simulink model "D53_LKAS"  (R2018b)
settings: Solver=ode3  StartTime=0.0  StopTime=10.0  FixedStep=0.01  RelTol=1e-3  EnableMultiTasking=on
model workspace (MAT data in the model file):
  MCOS : class17 (value not decoded)
  MCOS : class17 (value not decoded)
  MCOS : class17 (value not decoded)
  MCOS : class17 (value not decoded)
  MCOS : class17 (value not decoded)
  MCOS : class17 (value not decoded)
  MCOS : class17 (value not decoded)
  MCOS : class17 (value not decoded)
  MCOS : class17 (value not decoded)
  MCOS : class17 (value not decoded)
  MCOS : class17 (value not decoded)
  MCOS : class17 (value not decoded)
  MCOS : class17 (value not decoded)
  MCOS : class17 (value not decoded)
  MCOS : class17 (value not decoded)
  MCOS : class17 (value not decoded)
  MCOS : class17 (value not decoded)
  MCOS : class17 (value not decoded)
  MCOS : class17 (value not decoded)
  MCOS : class17 (value not decoded)
  MCOS : class17 (value not decoded)
  MCOS : class17 (value not decoded)
  MCOS : class17 (value not decoded)
  MCOS : class17 (value not decoded)
  MCOS : class17 (value not decoded)
  MCOS : class17 (value not decoded)
  MCOS : class17 (value not decoded)
  MCOS : class17 (value not decoded)
  MCOS : class17 (value not decoded)
  MCOS : class17 (value not decoded)
  MCOS : class17 (value not decoded)
  MCOS : class17 (value not decoded)
  MCOS : class17 (value not decoded)
  MCOS : class17 (value not decoded)
  MCOS : class17 (value not decoded)
  MCOS : class17 (value not decoded)
  MCOS : class17 (value not decoded)
  MCOS : class17 (value not decoded)
  MCOS : class17 (value not decoded)
  MCOS : class17 (value not decoded)
  MCOS : class17 (value not decoded)
  MCOS : class17 (value not decoded)
  MCOS : class17 (value not decoded)
  MCOS : class17 (value not decoded)
  MCOS : class17 (value not decoded)
  MCOS : class17 (value not decoded)
  MCOS : class17 (value not decoded)
  MCOS : class17 (value not decoded)
  MCOS : class17 (value not decoded)
  MCOS : class17 (value not decoded)
  MCOS : class17 (value not decoded)
  MCOS : class17 (value not decoded)
  MCOS : class17 (value not decoded)
  MCOS : class17 (value not decoded)
  MCOS : class17 (value not decoded)
  MCOS : class17 (value not decoded)
  MCOS : class17 (value not decoded)
  MCOS : class17 (value not decoded)
  MCOS : class17 (value not decoded)
  MCOS : class17 (value not decoded)
  MCOS : class17 (value not decoded)
  MCOS : class17 (value not decoded)
  MCOS : class17 (value not decoded)
  MCOS : class17 (value not decoded)
  MCOS : class17 (value not decoded)
  MCOS : class17 (value not decoded)
  MCOS : class17 (value not decoded)
  MCOS : class17 (value not decoded)
  MCOS : class17 (value not decoded)
  MCOS : class17 (value not decoded)
  MCOS : class17 (value not decoded)
  MCOS : class17 (value not decoded)
  MCOS : class17 (value not decoded)
  MCOS : class17 (value not decoded)
  MCOS : class17 (value not decoded)
  MCOS : class17 (value not decoded)
  MCOS : class17 (value not decoded)
  MCOS : class17 (value not decoded)
  MCOS : class17 (value not decoded)
  MCOS : class17 (value not decoded)
  MCOS : class17 (value not decoded)
  MCOS : class17 (value not decoded)
  MCOS : class17 (value not decoded)
  MCOS : class17 (value not decoded)
  MCOS : class17 (value not decoded)
  MCOS : class17 (value not decoded)
  MCOS : class17 (value not decoded)
  MCOS : class17 (value not decoded)
  MCOS : class17 (value not decoded)
values from neighbouring files (symbols this model uses):
  C = who    [Data_Made_Data.m]    (also in Data_Make_Data.m; Data_Process.m)
  LKA_SampleTime = Simulink.Parameter    [Model_NoProtect_Script.m]
  Monitor = find_system(strcat(filename,'/CAN Monitor (CANMon)/Monitor'),'SearchDepth',1,'BlockType','From')    [UpdateMon.m]    (also in UpdateMonAuto.m = find_system(strcat(scriptfile,'/CAN Monitor (CANMon)/Monitor; UpdateMonMdb.m; Update_MonAuto.m = find_system(strcat(scriptfile,'/CAN Monitor (CANMon)/Monitor; Update_MonMdb.m)
undefined symbols (not defined in the file or in its folder): LKA_CarWidth, LKA_StrRatio_C, LKA_Veh2CamL_C, LKA_Veh2CamW_C, LKA_WhlBaseL_C, LL_CompSWA_C, LL_CrvtPrvwT_C, LL_DesDvt_C, LL_DvtComp_C, LL_DvtPrvwT_C, LL_DvtSpdDet_vDvtSpdMin_C, LL_HdAgExT_C, LL_HdAgPrvwT_C, LL_LAccMax_C, LL_LAccRMax_C, LL_LDW_EarliestWarnLine_C, LL_LDW_LatestWarnLine_C, LL_LDWS_SUPPRESS_HEADING, LL_LFClb_TFC_DiffCtlBalance, LL_LFClb_TFC_DiffCtrlMaxSWA, LL_LFClb_TFC_DiffCtrlRatio, LL_LFClb_TFC_facmGainLutGain1_C, LL_LFClb_TFC_facmGainLutGain2_C, LL_LFClb_TFC_facmIntegRatio, LL_LFClb_TFC_facmKlat_C, LL_LFClb_TFC_FfCtlRatio_C, LL_LFClb_TFC_phiIntegCtlMaxSWA_C, LL_LFClb_TFC_tiKlatPrvwT_C, LL_LFClb_TFC_vGainLutVehSpdLwr_C, LL_LFClb_TFC_vGainLutVehSpdUpr_C, LL_LKA_EarliestWarnLine_C, LL_LKA_LatestWarnLine_C, LL_LKAExPrcs_ExitC0Dvt, LL_LKAExPrcs_ExitC0Swt, LL_LKAExPrcs_tiExitTime1, LL_LKAExPrcs_tiExitTime2, LL_LKAExPrcs_tiExitTime3, LL_LKAS_OUT_OF_CONTROL_LAT_VEL, LL_LKAS_OUT_OF_CONTROL_TTLC, LL_LKASWASyn_M0, LL_LKASWASyn_M1, LL_LKASWASyn_M2, LL_LKASWASyn_M3K, LL_LKASWASyn_SWAaddMax, LL_LKASWASyn_T2, LL_LKASWASyn_tiTrqSwaRtTime, LL_LKASWASyn_tiTrqSwaTime, LL_LKASWASyn_TrqMax, LL_LKASWASyn_TrqSwaAddSwt, LL_LKASWASyn_TrqSwaRateDiff, LL_LSpdCompT_C, LL_lStpLngth_C, LL_MAX_DELAY_EPSSTAR_TIME, LL_MAX_DRIVER_TORQUE_DISABLE, LL_MAX_DRIVER_TORQUE_ENABLE, LL_MAX_LANE_WIDTH_DISABLE, LL_MAX_LANE_WIDTH_ENABLE, LL_MAX_LAT_ACC_DISABLE, LL_MAX_LAT_ACC_ENABLE, LL_MAX_LDWS_SPEED_DISABLE ... (+29)
libraries: simulink x134, canmsglib x36, dspstat3 x3, simulink_extras x1
(part 11 of 17)

== system D53_LKAS/LL/LLOn/LKA/LKA Motion Planning (LKAMP) /Motion Planning Input Processing (MPInP)/Lane Information Selection (LaneInfoSel) ==
  LaneInfoSel_stLKAActvFlg : Inport
  LaneInfoSel_facmLftLane : Inport  Port=2
  LaneInfoSel_facmRgtLane : Inport  Port=3
  If : If  IfExpression=u1==1  ElseIfExpressions=u1==2
  If Action Subsystem1 : Subsystem  TreatAsAtomicUnit=on
  If Action Subsystem2 : Subsystem  TreatAsAtomicUnit=on
  If Action Subsystem3 : Subsystem  TreatAsAtomicUnit=on
  Merge : Merge  Inputs=3
  LaneInfoSel_facmActvLane : Outport
  wires:
  If/3 -> If Action Subsystem3/Action
  If Action Subsystem3/1(Out1) -> Merge/3
  If Action Subsystem1/1(Out1) -> Merge/2
  If/2 -> If Action Subsystem1/Action
  Merge/1 -> LaneInfoSel_facmActvLane/1
  If Action Subsystem2/1(Out1) -> Merge/1
  If/1 -> If Action Subsystem2/Action
  LaneInfoSel_stLKAActvFlg/1 -> If/1
  LaneInfoSel_facmLftLane/1 -> If Action Subsystem2/1(In1)
  LaneInfoSel_facmRgtLane/1 -> If Action Subsystem1/1(In1)

== system D53_LKAS/LL/LLOn/LKA/LKA Motion Planning (LKAMP) /Motion Planning Input Processing (MPInP)/Signal Latching2 ==
  In : Inport
  Add : Sum  OutDataTypeStr=uint16
  Constant : Constant  OutDataTypeStr=uint16  SampleTime=-1
  Constant2 : Constant  Value=LatchTime  OutDataTypeStr=uint16  SampleTime=-1
  If : If  NumInputs=2  IfExpression=u1==u2  ShowElse=off
  Memory : Memory  InheritSampleTime=on
  Saturation1 : Saturate  UpperLimit=10000  LowerLimit=0  OutDataTypeStr=uint16
  "if action " : Subsystem  TreatAsAtomicUnit=on
  Out : Outport
  wires:
  Saturation1/1 -> If/1, Memory/1
  Memory/1 -> Add/2
  Add/1 -> Saturation1/1
  Constant/1 -> Add/1
  If/1 -> "if action "/Action
  "if action "/1(Out) -> Out/1
  In/1 -> "if action "/1(In)
  Constant2/1 -> If/2

== system D53_LKAS/LL/LLOn/LKA/LKA Motion Planning (LKAMP) /Motion Planning Input Processing (MPInP)/Signal Latching3 ==
  In : Inport
  Add : Sum  OutDataTypeStr=uint16
  Constant : Constant  OutDataTypeStr=uint16  SampleTime=-1
  Constant2 : Constant  Value=LatchTime  OutDataTypeStr=uint16  SampleTime=-1
  If : If  NumInputs=2  IfExpression=u1==u2  ShowElse=off
  Memory : Memory  InheritSampleTime=on
  Saturation1 : Saturate  UpperLimit=10000  LowerLimit=0  OutDataTypeStr=uint16
  "if action " : Subsystem  TreatAsAtomicUnit=on
  Out : Outport
  wires:
  Constant2/1 -> If/2
  In/1 -> "if action "/1(In)
  "if action "/1(Out) -> Out/1
  If/1 -> "if action "/Action
  Constant/1 -> Add/1
  Add/1 -> Saturation1/1
  Memory/1 -> Add/2
  Saturation1/1 -> Memory/1, If/1

== system D53_LKAS/LL/LLOn/LKA/LKA Motion Planning (LKAMP) /Motion Planning Input Processing (MPInP)/Signal Latching4 ==
  In : Inport
  Add : Sum  OutDataTypeStr=uint16
  Constant : Constant  OutDataTypeStr=uint16  SampleTime=-1
  Constant2 : Constant  Value=LatchTime  OutDataTypeStr=uint16  SampleTime=-1
  If : If  NumInputs=2  IfExpression=u1==u2  ShowElse=off
  Memory : Memory  InheritSampleTime=on
  Saturation1 : Saturate  UpperLimit=10000  LowerLimit=0  OutDataTypeStr=uint16
  "if action " : Subsystem  TreatAsAtomicUnit=on
  Out : Outport
  wires:
  Saturation1/1 -> If/1, Memory/1
  Memory/1 -> Add/2
  Add/1 -> Saturation1/1
  Constant/1 -> Add/1
  If/1 -> "if action "/Action
  "if action "/1(Out) -> Out/1
  In/1 -> "if action "/1(In)
  Constant2/1 -> If/2

== system D53_LKAS/LL/LLOn/LKA/LKA Motion Planning (LKAMP) /Motion Planning Input Processing (MPInP)/Signal Latching5 ==
  In : Inport
  Add : Sum  OutDataTypeStr=uint16
  Constant : Constant  OutDataTypeStr=uint16  SampleTime=-1
  Constant2 : Constant  Value=LatchTime  OutDataTypeStr=uint16  SampleTime=-1
  If : If  NumInputs=2  IfExpression=u1==u2  ShowElse=off
  Memory : Memory  InheritSampleTime=on
  Saturation1 : Saturate  UpperLimit=10000  LowerLimit=0  OutDataTypeStr=uint16
  "if action " : Subsystem  TreatAsAtomicUnit=on
  Out : Outport
  wires:
  Saturation1/1 -> If/1, Memory/1
  Memory/1 -> Add/2
  Add/1 -> Saturation1/1
  Constant/1 -> Add/1
  If/1 -> "if action "/Action
  "if action "/1(Out) -> Out/1
  In/1 -> "if action "/1(In)
  Constant2/1 -> If/2

== system D53_LKAS/LL/LLOn/LKA/LKA Motion Planning (LKAMP) /Motion Planning Input Processing (MPInP)/Signal Latching6 ==
  In : Inport
  Add : Sum  OutDataTypeStr=uint16
  Constant : Constant  OutDataTypeStr=uint16  SampleTime=-1
  Constant2 : Constant  Value=LatchTime  OutDataTypeStr=uint16  SampleTime=-1
  If : If  NumInputs=2  IfExpression=u1==u2  ShowElse=off
  Memory : Memory  InheritSampleTime=on
  Saturation1 : Saturate  UpperLimit=10000  LowerLimit=0  OutDataTypeStr=uint16
  "if action " : Subsystem  TreatAsAtomicUnit=on
  Out : Outport
  wires:
  Saturation1/1 -> If/1, Memory/1
  Memory/1 -> Add/2
  Add/1 -> Saturation1/1
  Constant/1 -> Add/1
  If/1 -> "if action "/Action
  "if action "/1(Out) -> Out/1
  In/1 -> "if action "/1(In)
  Constant2/1 -> If/2

== system D53_LKAS/LL/LLOn/LKA/LKA Motion Planning (LKAMP) /Motion Planning Input Processing (MPInP)/Signal Latching7 ==
  In : Inport
  Add : Sum  OutDataTypeStr=uint16
  Constant : Constant  OutDataTypeStr=uint16  SampleTime=-1
  Constant2 : Constant  Value=LatchTime  OutDataTypeStr=uint16  SampleTime=-1
  If : If  NumInputs=2  IfExpression=u1==u2  ShowElse=off
  Memory : Memory  InheritSampleTime=on
  Saturation1 : Saturate  UpperLimit=10000  LowerLimit=0  OutDataTypeStr=uint16
  "if action " : Subsystem  TreatAsAtomicUnit=on
  Out : Outport
  wires:
  Constant2/1 -> If/2
  In/1 -> "if action "/1(In)
  "if action "/1(Out) -> Out/1
  If/1 -> "if action "/Action
  Constant/1 -> Add/1
  Add/1 -> Saturation1/1
  Memory/1 -> Add/2
  Saturation1/1 -> Memory/1, If/1

== system D53_LKAS/LL/LLOn/LKA/LKA Motion Planning (LKAMP) /Motion Planning Input Processing (MPInP)/Subsystem ==
  In1 : Inport
  If : If  IfExpression=u1==1  ElseIfExpressions=u1==2
  If Action Subsystem1 : Subsystem  TreatAsAtomicUnit=on
  If Action Subsystem2 : Subsystem  TreatAsAtomicUnit=on
  If Action Subsystem3 : Subsystem  TreatAsAtomicUnit=on
  Merge : Merge  Inputs=3
  Out6 : Outport
  wires:
  In1/1 -> If/1
  If/1 -> If Action Subsystem2/Action
  If Action Subsystem2/1(Out1) -> Merge/1
  Merge/1 -> Out6/1
  If/2 -> If Action Subsystem1/Action
  If Action Subsystem1/1(Out1) -> Merge/2
  If Action Subsystem3/1(Out1) -> Merge/3
  If/3 -> If Action Subsystem3/Action

== system D53_LKAS/LL/LLOn/LKA/LKA Motion Planning (LKAMP) /Switching Condition (SwtCon)/Ending Heading Angle Determination (EndHdAgDet) ==
  EndHdAgDet_stLKAActvFlg : Inport
  EndHdAgDet_vVehSpd : Inport  Port=2
  EndHdAgDet_crPrvwCrvt : Inport  Port=3
  EndHdAgDet_lLaneWidth_C : Inport  Port=4
  EndHdAgDet_lCarWidth_C : Inport  Port=5
  EndHdAgDet_tiHdAgExTime_C : Inport  Port=6
  EndHdAgDet_tiLSpdCompT_C : Inport  Port=7
  Add : Sum  Inputs=+-  OutDataTypeStr=single
  Add1 : Sum  OutDataTypeStr=single
  Divide : Product  Inputs=/*  OutDataTypeStr=single
  Divide1 : Product  Inputs=*/  OutDataTypeStr=single
  Lateral Speed Compensation (LSpdComp) : Subsystem
  kph To mps : Gain  Gain=1/3.6  OutDataTypeStr=single
  EndHdAgDet_phiHdAgMax : Outport
  wires:
  Divide/1 -> Divide1/1
  EndHdAgDet_lLaneWidth_C/1 -> Add/1
  EndHdAgDet_lCarWidth_C/1 -> Add/2
  kph To mps/1 -> Lateral Speed Compensation (LSpdComp)/1(LSpdComp_vVehSpd), Divide1/2
  EndHdAgDet_tiHdAgExTime_C/1 -> Divide/1
  EndHdAgDet_vVehSpd/1 -> kph To mps/1
  EndHdAgDet_stLKAActvFlg/1 -> Lateral Speed Compensation (LSpdComp)/2(LSpdComp_stLKAFlg)
  Add/1 -> Divide/2
  Lateral Speed Compensation (LSpdComp)/1(LSpdComp_phiLSpdComp) -> Add1/2
  Divide1/1 -> Add1/1
  Add1/1 -> EndHdAgDet_phiHdAgMax/1
  EndHdAgDet_crPrvwCrvt/1 -> Lateral Speed Compensation (LSpdComp)/3(LSpdComp_crPrvwCrvt)
  EndHdAgDet_tiLSpdCompT_C/1 -> Lateral Speed Compensation (LSpdComp)/4(LSpdComp_tiLSpdCompT_C)

== system D53_LKAS/LL/LLOn/LKA/LKA Motion Planning (LKAMP) /Switching Condition (SwtCon)/If Action Subsystem ==
  In1 : Inport
  Action Port : ActionPort  InitializeStates=reset
  Gain2 : Gain  Gain=-1  OutDataTypeStr=Inherit: Same as input
  Out1 : Outport
  wires:
  Gain2/1 -> Out1/1  "HdAgMax"
  In1/1 -> Gain2/1

== system D53_LKAS/LL/LLOn/LKA/LKA Motion Planning (LKAMP) /Switching Condition (SwtCon)/If Action Subsystem1 ==
  In1 : Inport
  Action Port : ActionPort  InitializeStates=reset
  Cast To Single1 : DataTypeConversion  LockScale=on
  Out1 : Outport
  wires:
  Cast To Single1/1 -> Out1/1  "HdAgMax"
  In1/1 -> Cast To Single1/1

== system D53_LKAS/LL/LLOn/LKA/LKA Motion Planning (LKAMP) /Switching Condition (SwtCon)/If Action Subsystem2 ==
  Action Port : ActionPort  InitializeStates=reset
  Constant2 : Constant  Value=0  OutDataTypeStr=single  SampleTime=-1
  Out1 : Outport
  wires:
  Constant2/1 -> Out1/1  "HdAgMax"

== system D53_LKAS/LL/LLOn/LKA/LKA Motion Planning (LKAMP) /Switching Condition (SwtCon)/Signal Latching ==
  In : Inport
  Add : Sum  OutDataTypeStr=uint16
  Constant : Constant  OutDataTypeStr=uint16  SampleTime=-1
  Constant2 : Constant  Value=LatchTime  OutDataTypeStr=uint16  SampleTime=-1
  If : If  NumInputs=2  IfExpression=u1==u2  ShowElse=off
  Memory : Memory  InheritSampleTime=on
  Saturation1 : Saturate  UpperLimit=10000  LowerLimit=0  OutDataTypeStr=uint16
  "if action " : Subsystem  TreatAsAtomicUnit=on
  Out : Outport
  wires:
  Saturation1/1 -> If/1
  Memory/1 -> Add/2
  Add/1 -> Saturation1/1, Memory/1
  Constant/1 -> Add/1
  If/1 -> "if action "/Action
  "if action "/1(Out) -> Out/1
  In/1 -> "if action "/1(In)
  Constant2/1 -> If/2

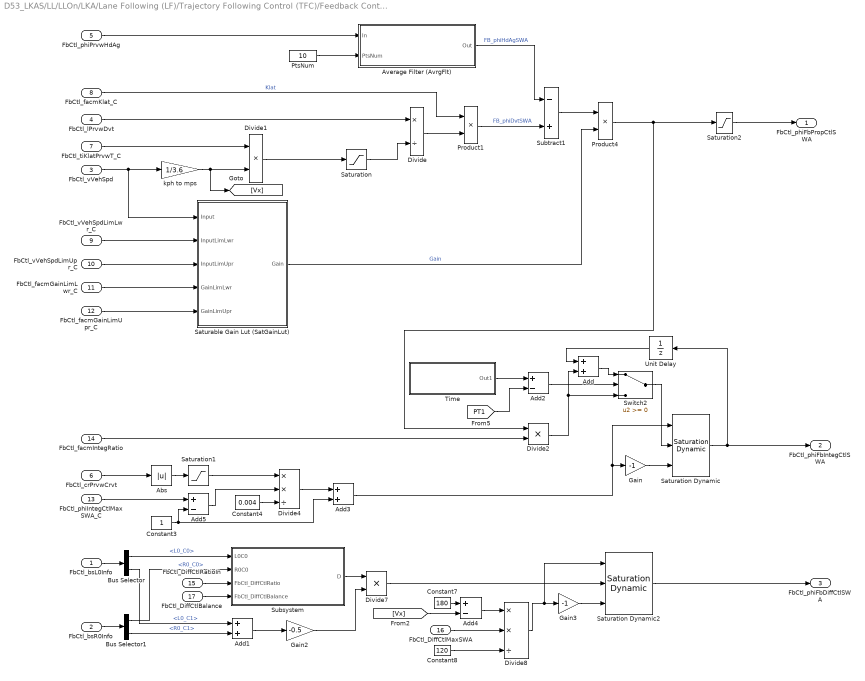
== system D53_LKAS/LL/LLOn/LKA/Lane Following (LF)/Trajectory Following Control (TFC)/Feedback Control (FbCtl) ==
  FbCtl_bsL0Info : Inport
  FbCtl_bsR0Info : Inport  Port=2
  FbCtl_vVehSpd : Inport  Port=3
  FbCtl_lPrvwDvt : Inport  Port=4
  FbCtl_phiPrvwHdAg : Inport  Port=5
  FbCtl_crPrvwCrvt : Inport  Port=6
  FbCtl_tiKlatPrvwT_C : Inport  Port=7
  FbCtl_facmKlat_C : Inport  Port=8
  FbCtl_vVehSpdLimLwr_C : Inport  Port=9
  FbCtl_vVehSpdLimUpr_C : Inport  Port=10
  FbCtl_facmGainLimLwr_C : Inport  Port=11
  FbCtl_facmGainLimUpr_C : Inport  Port=12
  FbCtl_phiIntegCtlMaxSWA_C : Inport  Port=13
  FbCtl_facmIntegRatio : Inport  Port=14
  FbCtl_DiffCtlRatioIn : Inport  Port=15
  FbCtl_DiffCtlMaxSWA : Inport  Port=16
  FbCtl_DiffCtlBalance : Inport  Port=17
  Abs : Abs
  Add : Sum
  Add1 : Sum
  Add2 : Sum  Inputs=+-
  Add3 : Sum
  Add4 : Sum  Inputs=+-
  Add5 : Sum  Inputs=+-
  Average Filter (AvrgFlt) : Subsystem
      mask Display:
      | port_label('input', 1, 'In');
      | port_label('input', 2, 'PtsNum');
      | port_label('output', 1, 'Out');
      | color('blue');
      | text(0.98,0.9,'VCDC Block','horizontalAlignment','right');
      | color('black');
      | text(0.5,0.55,'Average Filter','horizontalAlignment','center');
      | text(0.5,0.4,'(AvrgFlt)','horizontalAlignment','center');
  Bus Selector : BusSelector  OutputSignals=L0_C0,L0_C1
  Bus Selector1 : BusSelector  OutputSignals=R0_C0,R0_C1
  Constant3 : Constant  OutDataTypeStr=single
  Constant4 : Constant  Value=0.004  OutDataTypeStr=single
  Constant7 : Constant  Value=180  OutDataTypeStr=single
  Constant8 : Constant  Value=120  OutDataTypeStr=single
  Divide : Product  Inputs=*/
  Divide1 : Product  Inputs=**
  Divide2 : Product  Inputs=**
  Divide4 : Product  Inputs=**/
  Divide7 : Product  Inputs=**
  Divide8 : Product  Inputs=**/
  Gain : Gain  Gain=-1  OutDataTypeStr=single
  Gain2 : Gain  Gain=-0.5
  Gain3 : Gain  Gain=-1  OutDataTypeStr=single
  Product1 : Product  OutDataTypeStr=single  RndMeth=Zero
  Product4 : Product  OutDataTypeStr=single  RndMeth=Zero
  PtsNum : Constant  Value=10  OutDataTypeStr=single
  Saturable Gain Lut (SatGainLut) : MATLAB Function  TreatAsAtomicUnit=on
  Saturation : Saturate  UpperLimit=40  LowerLimit=5
  Saturation Dynamic : simulink/Discontinuities/Saturation Dynamic  OutMin=[]  OutMax=[]  OutDataTypeStr=Inherit: Same as second input  OutDataType=fixdt(1, 16)  OutScaling=2^-10  DoSatur=off
  Saturation Dynamic2 : simulink/Discontinuities/Saturation Dynamic  OutMin=[]  OutMax=[]  OutDataTypeStr=Inherit: Same as second input  OutDataType=fixdt(1, 16)  OutScaling=2^-10  DoSatur=off
  Saturation1 : Saturate  UpperLimit=0.004  LowerLimit=0.00001
  Saturation2 : Saturate  UpperLimit=360  LowerLimit=-360  OutDataTypeStr=single
  Subsystem : Subsystem
  Subtract1 : Sum  Inputs=-+
  Switch2 : Switch
  Time : Subsystem
      mask Display:
      | port_label('output', 1, 'TTime');
      | color('blue');
      | text(0.98,0.9,'VCDC Block','horizontalAlignment','right');
      | color('black');
      | text(0.5,0.55,'Tick Time','horizontalAlignment','center');
      | text(0.5,0.4,'(TTime)','horizontalAlignment','center');
  Unit Delay : UnitDelay  SampleTime=-1
  kph to mps : Gain  Gain=1/3.6  OutDataTypeStr=single
  FbCtl_phiFbPropCtlSWA : Outport
  FbCtl_phiFbIntegCtlSWA : Outport  Port=2
  FbCtl_phiFbDiffCtlSWA : Outport  Port=3
  wires:
  FbCtl_DiffCtlBalance/1 -> Subsystem/4(FbCtl_DiffCtlBalance)
  Add5/1 -> Divide4/2
  Constant4/1 -> Divide4/3
  Divide4/1 -> Add3/1
  Saturation1/1 -> Divide4/1
  Constant3/1 -> Add3/2, Add5/2
  Abs/1 -> Saturation1/1
  FbCtl_crPrvwCrvt/1 -> Abs/1
  Add/1 -> Switch2/1
  Switch2/1 -> Saturation Dynamic/2
  Add2/1 -> Switch2/2
  [PT1] -> Add2/2
  Time/1(Out1) -> Add2/1
  Saturation Dynamic2/1 -> FbCtl_phiFbDiffCtlSWA/1
  FbCtl_DiffCtlRatioIn/1 -> Subsystem/3(FbCtl_DiffCtlRatio)
  Subsystem/1(D) -> Divide7/1
  Bus Selector1/2 -> Add1/2  "<R0_C1>"
  Add1/1 -> Gain2/1
  Bus Selector/2 -> Add1/1  "<L0_C1>"
  [Vx] -> Add4/2
  Constant8/1 -> Divide8/3
  Add4/1 -> Divide8/1
  Constant7/1 -> Add4/1
  FbCtl_DiffCtlMaxSWA/1 -> Divide8/2
  Divide8/1 -> Saturation Dynamic2/1, Gain3/1
  Gain3/1 -> Saturation Dynamic2/3
  Divide7/1 -> Saturation Dynamic2/2
  Saturation Dynamic/1 -> Unit Delay/1, FbCtl_phiFbIntegCtlSWA/1
  Gain/1 -> Saturation Dynamic/3
  Unit Delay/1 -> Add/1
  FbCtl_vVehSpd/1 -> Saturable Gain Lut (SatGainLut)/1(Input), kph to mps/1
  FbCtl_phiIntegCtlMaxSWA_C/1 -> Add5/1
  Add3/1 -> Gain/1, Saturation Dynamic/1
  Subtract1/1 -> Product4/1
  Divide2/1 -> Switch2/3, Add/2
  FbCtl_facmIntegRatio/1 -> Divide2/2
  FbCtl_facmGainLimUpr_C/1 -> Saturable Gain Lut (SatGainLut)/5(GainLimUpr)
  FbCtl_facmGainLimLwr_C/1 -> Saturable Gain Lut (SatGainLut)/4(GainLimLwr)
  FbCtl_vVehSpdLimUpr_C/1 -> Saturable Gain Lut (SatGainLut)/3(InputLimUpr)
  FbCtl_vVehSpdLimLwr_C/1 -> Saturable Gain Lut (SatGainLut)/2(InputLimLwr)
  kph to mps/1 -> [Vx], Divide1/2
  Product4/1 -> Saturation2/1, Divide2/1
  FbCtl_phiPrvwHdAg/1 -> Average Filter (AvrgFlt)/1(In)
  Divide/1 -> Product1/2
  FbCtl_lPrvwDvt/1 -> Divide/1
  FbCtl_tiKlatPrvwT_C/1 -> Divide1/1
  Divide1/1 -> Saturation/1
  Saturation/1 -> Divide/2
  Saturation2/1 -> FbCtl_phiFbPropCtlSWA/1
  Saturable Gain Lut (SatGainLut)/1(Gain) -> Product4/2  "Gain"
  Average Filter (AvrgFlt)/1(Out) -> Subtract1/1  "FB_phiHdAgSWA"
  Product1/1 -> Subtract1/2  "FB_phiDvtSWA"
  FbCtl_facmKlat_C/1 -> Product1/1  "Klat"
  PtsNum/1 -> Average Filter (AvrgFlt)/2(PtsNum)
  FbCtl_bsL0Info/1 -> Bus Selector/1
  FbCtl_bsR0Info/1 -> Bus Selector1/1
  Bus Selector/1 -> Subsystem/1(L0C0)  "<L0_C0>"
  Bus Selector1/1 -> Subsystem/2(R0C0)  "<R0_C0>"
  Gain2/1 -> Divide7/2

== system D53_LKAS/LL/LLOn/LKA/Lane Following (LF)/Trajectory Following Control (TFC)/Feedforward Control (FfCtl) ==
  FfCtl_FfCtlRatio_C : Inport
  FfCtl_vVehSpd : Inport  Port=2
  FfCtl_crPrvwCrvt : Inport  Port=3
  FfCtl_lWhlBase_SY : Inport  Port=4
  FfCtl_rTraRatio_C : Inport  Port=5
  Add : Sum  OutDataTypeStr=single
  Constant1 : Constant  OutDataTypeStr=single
  Divide : Product  Inputs=*/  OutDataTypeStr=single
  Divide1 : Product  Inputs=*/  OutDataTypeStr=single
  Gain2 : Gain  Gain=-1  OutDataTypeStr=single
  Lookup Table2 : Lookup_n-D  NumberOfTableDimensions=1  BreakpointsForDimension1=[11.7,18.83,26.98,31.98,51.04,79,86.08,90.59]  BeginIndexSearchUsingPreviousIndexResult=on  Table=[0.012141,0.005179,0.00298,0.002547,0.001715,0.001283,0.001021,0.000982]  DiagnosticForOutOfRangeInput=Warning  RemoveProtectionInput=on  InternalRulePriority=Speed  OutDataTypeStr=single  InputSameDT=on
  Math Function : Math  Operator=magnitude^2  OutDataTypeStr=single  SaturateOnIntegerOverflow=on
  Product : Product  OutDataTypeStr=single
  Product1 : Product  OutDataTypeStr=single
  Product2 : Product  OutDataTypeStr=single
  Product3 : Product  Inputs=3  OutDataTypeStr=single
  Saturation1 : Saturate  UpperLimit=0.01  LowerLimit=0
  kph to mps : Gain  Gain=1/3.6  OutDataTypeStr=single
  rad to deg : Gain  Gain=180/pi  OutDataTypeStr=single
  FfCtl_phiFfSWA : Outport
  wires:
  Saturation1/1 -> Product2/2  "FfCtl_facmUSG_C"
  Lookup Table2/1 -> Saturation1/1
  FfCtl_FfCtlRatio_C/1 -> Product3/1
  FfCtl_rTraRatio_C/1 -> Product3/3
  Product3/1 -> Gain2/1
  FfCtl_vVehSpd/1 -> kph to mps/1, Lookup Table2/1
  FfCtl_crPrvwCrvt/1 -> Product/2
  Product/1 -> rad to deg/1
  Math Function/1 -> Product2/1
  Product2/1 -> Add/1
  Constant1/1 -> Add/2
  Add/1 -> Divide1/1
  FfCtl_lWhlBase_SY/1 -> Divide/2
  Divide/1 -> Divide1/2
  Divide1/1 -> Product1/2
  Product1/1 -> Product3/2
  rad to deg/1 -> Product1/1
  kph to mps/1 -> Product/1, Math Function/1, Divide/1
  Gain2/1 -> FfCtl_phiFfSWA/1

== system D53_LKAS/LL/LLOn/LKA/Plan To LaneFollowing (PTLF)/InsideJudge1/If Action Subsystem ==
  T1 : Inport
  Plan : Inport  Port=2
  HdAgLft : Inport  Port=3
  Time : Inport  Port=4
  Action Port : ActionPort  InitializeStates=reset
  Add : Sum
  Cast To Single : DataTypeConversion  OutDataTypeStr=uint8
  Compare To Constant : simulink/Logic and Bit Operations/Compare To Constant  relop=>=  const=0  OutDataTypeStr=boolean
  Detect Decrease : simulink/Logic and Bit Operations/Detect Decrease  vinit=0.0  OutDataTypeStr=boolean
  If Action Subsystem : Subsystem  TreatAsAtomicUnit=on
  If Action Subsystem2 : Subsystem  TreatAsAtomicUnit=on
  Logical Operator : Logic  AllPortsSameDT=off  OutDataTypeStr=boolean
  Memory : Memory  InheritSampleTime=on
  Relational Operator : RelationalOperator  OutDataTypeStr=boolean  RndMeth=Simplest
  Saturation : Saturate  UpperLimit=5  LowerLimit=0
  Switch : Switch  Criteria=u2 > Threshold
  Switch1 : Switch  Criteria=u2 > Threshold
  T1_1 : Outport
  Plan_1 : Outport  Port=2
  wires:
  Switch1/1 -> Plan_1/1
  Switch/1 -> T1_1/1
  If Action Subsystem2/2(Plan_1) -> Switch1/3
  If Action Subsystem2/1(T1_1) -> Switch/3
  If Action Subsystem/2(Plan_1) -> Switch1/1
  If Action Subsystem/1(T1_1) -> Switch/1
  Saturation/1 -> Memory/1, If Action Subsystem/Enable, Switch/2, Switch1/2
  Cast To Single/1 -> Add/1
  Logical Operator/1 -> Cast To Single/1
  Memory/1 -> Add/2
  Add/1 -> Saturation/1
  Relational Operator/1 -> Logical Operator/2
  Detect Decrease/1 -> Logical Operator/1
  T1/1 -> Relational Operator/1, If Action Subsystem2/1(T1)
  Plan/1 -> If Action Subsystem/2(Plan), If Action Subsystem2/2(Plan)
  Time/1 -> Relational Operator/2, If Action Subsystem/1(T1)
  Compare To Constant/1 -> Detect Decrease/1
  HdAgLft/1 -> Compare To Constant/1

== system D53_LKAS/LL/LLOn/LKA/Plan To LaneFollowing (PTLF)/InsideJudge1/If Action Subsystem1 ==
  T1 : Inport
  Plan : Inport  Port=2
  HdAgRgt : Inport  Port=3
  Time : Inport  Port=4
  Action Port : ActionPort  InitializeStates=reset
  Add : Sum
  Cast To Single : DataTypeConversion  OutDataTypeStr=uint8
  Compare To Constant : simulink/Logic and Bit Operations/Compare To Constant  relop=<=  const=0  OutDataTypeStr=boolean
  Detect Decrease : simulink/Logic and Bit Operations/Detect Decrease  vinit=0.0  OutDataTypeStr=boolean
  If Action Subsystem : Subsystem  TreatAsAtomicUnit=on
  If Action Subsystem2 : Subsystem  TreatAsAtomicUnit=on
  Logical Operator : Logic  AllPortsSameDT=off  OutDataTypeStr=boolean
  Memory : Memory  InheritSampleTime=on
  Relational Operator : RelationalOperator  OutDataTypeStr=boolean  RndMeth=Simplest
  Saturation : Saturate  UpperLimit=5  LowerLimit=0
  Switch : Switch  Criteria=u2 > Threshold
  Switch1 : Switch  Criteria=u2 > Threshold
  T1_1 : Outport
  Plan_1 : Outport  Port=2
  wires:
  Plan/1 -> If Action Subsystem2/2(Plan), If Action Subsystem/2(Plan)
  If Action Subsystem/1(T1_1) -> Switch/1
  If Action Subsystem2/2(Plan_1) -> Switch1/3
  Switch1/1 -> Plan_1/1
  Switch/1 -> T1_1/1
  If Action Subsystem/2(Plan_1) -> Switch1/1
  If Action Subsystem2/1(T1_1) -> Switch/3
  Saturation/1 -> If Action Subsystem/Enable, Switch/2, Switch1/2, Memory/1
  Cast To Single/1 -> Add/1
  Logical Operator/1 -> Cast To Single/1
  Memory/1 -> Add/2
  T1/1 -> Relational Operator/1, If Action Subsystem2/1(T1)
  Add/1 -> Saturation/1
  Time/1 -> If Action Subsystem/1(T1), Relational Operator/2
  HdAgRgt/1 -> Compare To Constant/1
  Compare To Constant/1 -> Detect Decrease/1
  Detect Decrease/1 -> Logical Operator/1
  Relational Operator/1 -> Logical Operator/2

== system D53_LKAS/LL/LLOn/LKA/Plan To LaneFollowing (PTLF)/InsideJudge1/If Action Subsystem2 ==
  T1 : Inport
  Plan : Inport  Port=2
  Action Port : ActionPort  InitializeStates=reset
  T1_1 : Outport
  Plan_1 : Outport  Port=2
  wires:
  Plan/1 -> Plan_1/1
  T1/1 -> T1_1/1

== system D53_LKAS/LL/LLOn/LKA Input Processing (LKAInP)/Predicted Deviation Calculation (PrDvt)/Lane Information Selection (LaneInfoSel)/If Action Subsystem1 ==
  In1 : Inport
  Action Port : ActionPort  InitializeStates=reset
  Out1 : Outport
  wires:
  In1/1 -> Out1/1

== system D53_LKAS/LL/LLOn/LKA Input Processing (LKAInP)/Predicted Deviation Calculation (PrDvt)/Lane Information Selection (LaneInfoSel)/If Action Subsystem2 ==
  In1 : Inport
  Action Port : ActionPort  InitializeStates=reset
  Out1 : Outport
  wires:
  In1/1 -> Out1/1

== system D53_LKAS/LL/LLOn/LKA Input Processing (LKAInP)/Predicted Deviation Calculation (PrDvt)/Lane Information Selection (LaneInfoSel)/If Action Subsystem3 ==
  In1 : Inport
  In2 : Inport  Port=2
  Action Port : ActionPort  InitializeStates=reset
  Add : Sum
  Gain : Gain  Gain=0.5
  Out1 : Outport
  wires:
  Add/1 -> Gain/1
  In2/1 -> Add/2
  In1/1 -> Add/1
  Gain/1 -> Out1/1

== system D53_LKAS/LL/LLOn/LKA Input Processing (LKAInP)/Predicted Deviation Calculation (PrDvt)/Lane Information Selection (LaneInfoSel)1/If Action Subsystem1 ==
  In1 : Inport
  Action Port : ActionPort  InitializeStates=reset
  Out1 : Outport
  wires:
  In1/1 -> Out1/1

== system D53_LKAS/LL/LLOn/LKA Input Processing (LKAInP)/Predicted Deviation Calculation (PrDvt)/Lane Information Selection (LaneInfoSel)1/If Action Subsystem2 ==
  In1 : Inport
  Action Port : ActionPort  InitializeStates=reset
  Out1 : Outport
  wires:
  In1/1 -> Out1/1

== system D53_LKAS/LL/LLOn/LKA Input Processing (LKAInP)/Predicted Deviation Calculation (PrDvt)/Lane Information Selection (LaneInfoSel)1/If Action Subsystem3 ==
  In1 : Inport
  In2 : Inport  Port=2
  Action Port : ActionPort  InitializeStates=reset
  Min : MinMax  Inputs=2
  Out1 : Outport
  wires:
  Min/1 -> Out1/1
  In1/1 -> Min/1
  In2/1 -> Min/2

== system D53_LKAS/LL/LLOn/LKA Input Processing (LKAInP)/Predicted Heading Angle Calculation (PrHdAg)/Lane Information Selection (LaneInfoSel)/If Action Subsystem1 ==
  In1 : Inport
  Action Port : ActionPort  InitializeStates=reset
  Out1 : Outport
  wires:
  In1/1 -> Out1/1

== system D53_LKAS/LL/LLOn/LKA Input Processing (LKAInP)/Predicted Heading Angle Calculation (PrHdAg)/Lane Information Selection (LaneInfoSel)/If Action Subsystem2 ==
  In1 : Inport
  Action Port : ActionPort  InitializeStates=reset
  Out1 : Outport
  wires:
  In1/1 -> Out1/1

== system D53_LKAS/LL/LLOn/LKA Input Processing (LKAInP)/Predicted Heading Angle Calculation (PrHdAg)/Lane Information Selection (LaneInfoSel)/If Action Subsystem3 ==
  In1 : Inport
  In2 : Inport  Port=2
  Action Port : ActionPort  InitializeStates=reset
  Add : Sum
  Gain : Gain  Gain=0.5
  Out1 : Outport
  wires:
  In2/1 -> Add/2
  In1/1 -> Add/1
  Add/1 -> Gain/1
  Gain/1 -> Out1/1

== system D53_LKAS/LL/LLOn/LKA Input Processing (LKAInP)/Predicted Heading Angle Calculation (PrHdAg)/Lane Information Selection (LaneInfoSel)1/If Action Subsystem1 ==
  In1 : Inport
  Action Port : ActionPort  InitializeStates=reset
  Out1 : Outport
  wires:
  In1/1 -> Out1/1

== system D53_LKAS/LL/LLOn/LKA Input Processing (LKAInP)/Predicted Heading Angle Calculation (PrHdAg)/Lane Information Selection (LaneInfoSel)1/If Action Subsystem2 ==
  In1 : Inport
  Action Port : ActionPort  InitializeStates=reset
  Out1 : Outport
  wires:
  In1/1 -> Out1/1

== system D53_LKAS/LL/LLOn/LKA Input Processing (LKAInP)/Predicted Heading Angle Calculation (PrHdAg)/Lane Information Selection (LaneInfoSel)1/If Action Subsystem3 ==
  In1 : Inport
  In2 : Inport  Port=2
  Action Port : ActionPort  InitializeStates=reset
  Add : Sum
  Gain : Gain  Gain=0.5
  Out1 : Outport
  wires:
  Gain/1 -> Out1/1
  Add/1 -> Gain/1
  In1/1 -> Add/1
  In2/1 -> Add/2

== system D53_LKAS/LL/LLOn/LKA Input Processing (LKAInP)/Predicted Heading Angle Calculation (PrHdAg)/Perdicted Heading Angle Compensation (PrdcHdAgComp)/Yaw Rate Stable Gain (YRSG) ==
  YRSG_vVehSpd : Inport
  Add : Sum  OutDataTypeStr=single
  Bus Selector : BusSelector  OutputSignals=LKA_WhlBaseL_C
  Divide2 : Product  Inputs=*/  OutDataTypeStr=single
  Divide3 : Product  Inputs=*/  OutDataTypeStr=single
  Lookup Table2 : Lookup_n-D  NumberOfTableDimensions=1  BreakpointsForDimension1=[11.7,18.83,26.98,31.98,51.04,79,86.08,90.59]  BeginIndexSearchUsingPreviousIndexResult=on  Table=[0.012141,0.005179,0.00298,0.002547,0.001715,0.001283,0.001021,0.000982]  DiagnosticForOutOfRangeInput=Warning  RemoveProtectionInput=on  InternalRulePriority=Speed  OutDataTypeStr=single  InputSameDT=on
  Product1 : Product  Inputs=3  OutDataTypeStr=single
  Saturation1 : Saturate  UpperLimit=0.012141  LowerLimit=0.000982
  "constant " : Constant  OutDataTypeStr=single
  kph To mps : Gain  Gain=1/3.6  OutDataTypeStr=single
  YRSG_dphiYRSG : Outport
  wires:
  [LLClb_bsConstantClb] -> Bus Selector/1
  YRSG_vVehSpd/1 -> kph To mps/1, Lookup Table2/1
  Bus Selector/1 -> Divide2/2  "<LKA_WhlBaseL_C>"
  Divide2/1 -> Divide3/1
  Product1/1 -> Add/1
  "constant "/1 -> Add/2
  Add/1 -> Divide3/2
  Divide3/1 -> YRSG_dphiYRSG/1
  Lookup Table2/1 -> Saturation1/1
  Saturation1/1 -> Product1/3
  kph To mps/1 -> Product1/2, Product1/1, Divide2/1

== system D53_LKAS/LL/LLOn/LKA Input Processing (LKAInP)/Previewed Curvature (PrCrvt)/Lane Information Selection (LaneInfoSel)/If Action Subsystem1 ==
  In1 : Inport
  Action Port : ActionPort  InitializeStates=reset
  Out1 : Outport
  wires:
  In1/1 -> Out1/1

== system D53_LKAS/LL/LLOn/LKA Input Processing (LKAInP)/Previewed Curvature (PrCrvt)/Lane Information Selection (LaneInfoSel)/If Action Subsystem2 ==
  In1 : Inport
  Action Port : ActionPort  InitializeStates=reset
  Out1 : Outport
  wires:
  In1/1 -> Out1/1

== system D53_LKAS/LL/LLOn/LKA Input Processing (LKAInP)/Previewed Curvature (PrCrvt)/Lane Information Selection (LaneInfoSel)/If Action Subsystem3 ==
  In1 : Inport
  In2 : Inport  Port=2
  Action Port : ActionPort  InitializeStates=reset
  Add : Sum
  Gain : Gain  Gain=0.5
  Out1 : Outport
  wires:
  Add/1 -> Gain/1
  In2/1 -> Add/2
  In1/1 -> Add/1
  Gain/1 -> Out1/1

== system D53_LKAS/LL/LLOn/LKA Input Processing (LKAInP)/Steering Wheel Position Calculation (SWAPosCal)/Subsystem/LowPass ==
  T : Inport
  u : Inport  Port=2
  dT : Inport  Port=3
  Add : Sum  Inputs=+-
  Add1 : Sum
  Add2 : Sum  OutDataTypeStr=single
  Divide : Product  Inputs=*/
  Divide1 : Product  Inputs=**
  Memory3 : Memory  InheritSampleTime=on
  SWACmdSyn_tiSmplT_C4 : Constant  OutDataTypeStr=single
  Saturation : Saturate  UpperLimit=50  LowerLimit=0
  Switch : Switch  Criteria=u2 > Threshold  Threshold=1
  Unit Delay : UnitDelay  SampleTime=-1
  y : Outport
  wires:
  T/1 -> Divide/2
  dT/1 -> Divide/1
  u/1 -> Switch/3, Add/1
  Divide/1 -> Divide1/1
  Add/1 -> Divide1/2
  Divide1/1 -> Add1/1
  Unit Delay/1 -> Add/2, Add1/2
  Add1/1 -> Switch/1
  SWACmdSyn_tiSmplT_C4/1 -> Add2/1
  Add2/1 -> Saturation/1
  Saturation/1 -> Switch/2, Memory3/1
  Memory3/1 -> Add2/2
  Switch/1 -> y/1, Unit Delay/1

== system D53_LKAS/LL/LLOn/LKA Input Processing (LKAInP)/Steering Wheel Position Calculation (SWAPosCal)/Subsystem1/Subsystem ==
  In : Inport
  In1 : Inport  Port=2
  Enable : EnablePort  StatesWhenEnabling=reset
  Add1 : Sum  OutDataTypeStr=uint16
  Cast To Single : DataTypeConversion  OutDataTypeStr=uint16
  Cast To Single1 : DataTypeConversion  OutDataTypeStr=uint16
  Memory : Memory  InheritSampleTime=on
  Relational Operator : RelationalOperator  OutDataTypeStr=boolean  RndMeth=Nearest
  Saturation : Saturate  UpperLimit=3000  LowerLimit=0  OutDataTypeStr=uint16
  Out : Outport  OutputWhenDisabled=reset  InitialOutput=0
  wires:
  Add1/1 -> Saturation/1
  Saturation/1 -> Memory/1, Relational Operator/1
  Memory/1 -> Add1/2
  Cast To Single/1 -> Add1/1
  In1/1 -> Cast To Single1/1
  Relational Operator/1 -> Out/1
  In/1 -> Cast To Single/1
  Cast To Single1/1 -> Relational Operator/2

== system D53_LKAS/LL/LLOn/LL State Determination (LLStateDet)/LL State Machine Conditions (LLSMCon)/Activation Condition (ActvC)/Activation Condition Synthesis (ActvCSyn) ==
  ActvCSyn_stDACMode : Inport
  ActvCSyn_stEPSCtlEC : Inport  Port=2
  ActvCSyn_stDvtThresActvFlgLDW : Inport  Port=3
  ActvCSyn_stDvtThresActvFlgLKA : Inport  Port=4
  ActvCSyn_stLaneQlECFlg : Inport  Port=5
  Default Flag (DflFlg) : Subsystem  TreatAsAtomicUnit=on
  Default Flag (DflFlg)1 : Subsystem  TreatAsAtomicUnit=on
  If : If  NumInputs=3  IfExpression=(u1 ==1|u1==2)& u2 == 1 & u3 == 1  ElseIfExpressions=(u1 ==1|u1==2)& u2 == 2 & u3 == 1
  If1 : If  NumInputs=4  IfExpression=u1 == 2 & u2 == 1 & u3 == 1 & u4 == 1  ElseIfExpressions=u1 == 2 & u2 == 2 & u3 == 1 & u4 == 1
  LDW Left Active Flag (LDWLftActvFlg) : Subsystem  TreatAsAtomicUnit=on
  LDW Right Active Flag (LDWRgtActvFlg) : Subsystem  TreatAsAtomicUnit=on
  LKA Left Active Flag (LKALftActvFlg)1 : Subsystem  TreatAsAtomicUnit=on
  LKA Right Active Flag (LKARgtActvFlg)1 : Subsystem  TreatAsAtomicUnit=on
  Merge : Merge  Inputs=3
  Merge2 : Merge  Inputs=3
  ActvCSyn_stLDWActvCSyn : Outport
  ActvCSyn_stLKAActvCSyn : Outport  Port=2
  wires:
  ActvCSyn_stDvtThresActvFlgLDW/1 -> If/2
  ActvCSyn_stLaneQlECFlg/1 -> If1/4, If/3
  ActvCSyn_stDvtThresActvFlgLKA/1 -> If1/2
  ActvCSyn_stEPSCtlEC/1 -> If1/3
  Default Flag (DflFlg)1/1(Out) -> Merge2/3
  If1/2 -> LKA Right Active Flag (LKARgtActvFlg)1/Action
  LKA Right Active Flag (LKARgtActvFlg)1/1(Out) -> Merge2/2
  If1/1 -> LKA Left Active Flag (LKALftActvFlg)1/Action
  LKA Left Active Flag (LKALftActvFlg)1/1(Out) -> Merge2/1
  Merge2/1 -> ActvCSyn_stLKAActvCSyn/1
  Default Flag (DflFlg)/1(Out) -> Merge/3
  If1/3 -> Default Flag (DflFlg)1/Action
  Merge/1 -> ActvCSyn_stLDWActvCSyn/1
  LDW Right Active Flag (LDWRgtActvFlg)/1(Out) -> Merge/2
  ActvCSyn_stDACMode/1 -> If/1, If1/1
  If/2 -> LDW Right Active Flag (LDWRgtActvFlg)/Action
  If/3 -> Default Flag (DflFlg)/Action
  If/1 -> LDW Left Active Flag (LDWLftActvFlg)/Action
  LDW Left Active Flag (LDWLftActvFlg)/1(Out) -> Merge/1

== system D53_LKAS/LL/LLOn/LL State Determination (LLStateDet)/LL State Machine Conditions (LLSMCon)/Activation Condition (ActvC)/Deviation Threshold Condition (DvtThresCon) ==
  DvtThresCon_vVehSpd : Inport
  DvtThresCon_bsL0Info : Inport  Port=2
  DvtThresCon_bsR0Info : Inport  Port=3
  DvtThresCon_bsTTLCInfo : Inport  Port=4
  DvtThresCon_bsHdAgInfo : Inport  Port=5
  DvtThresCon_bsDvtThresClb : Inport  Port=6
  Active Lane Calculation (ActLanCalc) : Subsystem
  Bus Selector : BusSelector  OutputSignals=LftTTLC,RgtTTLC
  Bus Selector1 : BusSelector  OutputSignals=ActvCClb
  Bus Selector2 : BusSelector  OutputSignals=phiHdAgLft,phiHdAgRgt
  Deviation Calculation (DvtCalc) : Subsystem
  Deviation Speed Calculation (DvtSpdCalc) : Subsystem
  Deviation Threshold Judgement LDW (DvtThresJdg) : Subsystem
  Deviation Threshold Judgement LKA (DvtThresJdg) : Subsystem
  Saturation1 : Saturate  UpperLimit=2  LowerLimit=-2
  Saturation5 : Saturate  UpperLimit=2  LowerLimit=-2
  DvtThresCon_stDvtThresActvFlgLDW : Outport
  DvtThresCon_stDvtThresActvFlgLKA : Outport  Port=2
  wires:
  Deviation Threshold Judgement LDW (DvtThresJdg)/1(DvtThresJdg_stDvtThresActvFlg) -> DvtThresCon_stDvtThresActvFlgLDW/1  "DvtThresActvFlg"
  Saturation1/1 -> Deviation Threshold Judgement LKA (DvtThresJdg)/2(DvtThresJdg_lRgtDvt), Deviation Threshold Judgement LDW (DvtThresJdg)/2(DvtThresJdg_lRgtDvt)
  Saturation5/1 -> Deviation Threshold Judgement LKA (DvtThresJdg)/1(DvtThresJdg_lLftDvt), Deviation Threshold Judgement LDW (DvtThresJdg)/1(DvtThresJdg_lLftDvt)
  Bus Selector2/2 -> Deviation Speed Calculation (DvtSpdCalc)/2(DvtSpdCalc_phiPrvwHdAgRgt)  "<phiHdAgRgt>"
  Bus Selector2/1 -> Deviation Speed Calculation (DvtSpdCalc)/1(DvtSpdCalc_phiPrvwHdAgLft)  "<phiHdAgLft>"
  DvtThresCon_bsHdAgInfo/1 -> Bus Selector2/1
  DvtThresCon_bsTTLCInfo/1 -> Bus Selector/1  "TTLCInfo"
  DvtThresCon_vVehSpd/1 -> Deviation Speed Calculation (DvtSpdCalc)/3(DvtSpdCalc_vVehSpd)
  Active Lane Calculation (ActLanCalc)/1(ActLanCalc_ActvCClbOut) -> Deviation Threshold Judgement LKA (DvtThresJdg)/7(DvtThresJdg_bsDvtThresClb), Deviation Threshold Judgement LDW (DvtThresJdg)/7(DvtThresJdg_bsDvtThresClb)
  DvtThresCon_bsDvtThresClb/1 -> Bus Selector1/1
  Deviation Threshold Judgement LKA (DvtThresJdg)/1(DvtThresJdg_stDvtThresActvFlg) -> DvtThresCon_stDvtThresActvFlgLKA/1  "DvtThresActvFlg"
  Bus Selector/2 -> Deviation Threshold Judgement LKA (DvtThresJdg)/6(DvtThresJdg_tiRgtTTLC), Deviation Threshold Judgement LDW (DvtThresJdg)/6(DvtThresJdg_tiRgtTTLC)  "<RgtTTLC>"
  Bus Selector/1 -> Deviation Threshold Judgement LKA (DvtThresJdg)/5(DvtThresJdg_tiLftTTLC), Deviation Threshold Judgement LDW (DvtThresJdg)/5(DvtThresJdg_tiLftTTLC)  "<LftTTLC>"
  Deviation Speed Calculation (DvtSpdCalc)/2(DvtSpdCalc_vRgtDvtSpd) -> Deviation Threshold Judgement LKA (DvtThresJdg)/4(DvtThresJdg_vRgtDvtSpd), Deviation Threshold Judgement LDW (DvtThresJdg)/4(DvtThresJdg_vRgtDvtSpd)  "DvtSpdCalc_vRgtDvtSpd"
  Deviation Speed Calculation (DvtSpdCalc)/1(DvtSpdCalc_vLftDvtSpd) -> Deviation Threshold Judgement LKA (DvtThresJdg)/3(DvtThresJdg_vLftDvtSpd), Deviation Threshold Judgement LDW (DvtThresJdg)/3(DvtThresJdg_vLftDvtSpd)  "DvtSpdCalc_vLftDvtSpd"
  Deviation Calculation (DvtCalc)/2(DvtCalc_lRgtDvt) -> Saturation1/1  "DvtCalc_lRgtDvt"
  Deviation Calculation (DvtCalc)/1(DvtCalc_lLftDvt) -> Saturation5/1  "DvtCalc_lLftDvt"
  DvtThresCon_bsR0Info/1 -> Active Lane Calculation (ActLanCalc)/2(ActLanCalc_bsR0Info), Deviation Calculation (DvtCalc)/2(DvtCalc_bsR0Info)
  DvtThresCon_bsL0Info/1 -> Active Lane Calculation (ActLanCalc)/1(ActLanCalc_bsL0Info), Deviation Calculation (DvtCalc)/1(DvtCalc_bsL0Info)
  Bus Selector1/1 -> Active Lane Calculation (ActLanCalc)/3(ActLanCalc_ActvCClb)  "<ActvCClb>"

== system D53_LKAS/LL/LLOn/LL State Determination (LLStateDet)/LL State Machine Conditions (LLSMCon)/Activation Condition (ActvC)/EPS Controllability Enable Condition (EPSCtlEC) ==
  EPSCtlEC_bsEPSInfo : Inport
  Bus Selector : BusSelector  OutputSignals=EPS_LKA_State
  Cast To Single : DataTypeConversion  OutDataTypeStr=uint8
  Compare To Constant : simulink/Logic and Bit Operations/Compare To Constant  relop===  const=1  OutDataTypeStr=boolean
  Compare To Constant1 : simulink/Logic and Bit Operations/Compare To Constant  relop===  const=3  OutDataTypeStr=boolean
  Logical Operator : Logic  Operator=OR  AllPortsSameDT=off  OutDataTypeStr=boolean
  EPSCtlEC_stEPSCtlEC : Outport
  wires:
  Cast To Single/1 -> EPSCtlEC_stEPSCtlEC/1
  Compare To Constant/1 -> Logical Operator/1
  Bus Selector/1 -> Compare To Constant/1, Compare To Constant1/1  "<EPS_LKA_State>"
  EPSCtlEC_bsEPSInfo/1 -> Bus Selector/1
  Compare To Constant1/1 -> Logical Operator/2
  Logical Operator/1 -> Cast To Single/1

== system D53_LKAS/LL/LLOn/LL State Determination (LLStateDet)/LL State Machine Conditions (LLSMCon)/Activation Condition (ActvC)/Lane Quality Enable Condition (LaneQlEC) ==
  LaneQlEC_stDvtThresActvFlg : Inport
  LaneQlEC_stFacmL0Ql : Inport  Port=2
  LaneQlEC_stFacmR0Ql : Inport  Port=3
  Compare To Constant : simulink/Logic and Bit Operations/Compare To Constant  relop=>  const=2  OutDataTypeStr=boolean
  Compare To Constant1 : simulink/Logic and Bit Operations/Compare To Constant  relop=>  const=2  OutDataTypeStr=boolean
  Compare To Constant2 : simulink/Logic and Bit Operations/Compare To Constant  relop===  const=2  OutDataTypeStr=boolean
  Compare To Constant3 : simulink/Logic and Bit Operations/Compare To Constant  relop===  const=1  OutDataTypeStr=boolean
  Data Type Conversion : DataTypeConversion  OutDataTypeStr=uint8
  Logical Operator : Logic  AllPortsSameDT=off  OutDataTypeStr=boolean
  Logical Operator1 : Logic  AllPortsSameDT=off  OutDataTypeStr=boolean
  Logical Operator2 : Logic  Operator=OR  AllPortsSameDT=off  OutDataTypeStr=boolean
  LaneQlEC_stLaneQlECFlgLKA : Outport
  wires:
  Logical Operator2/1 -> Data Type Conversion/1
  Logical Operator1/1 -> Logical Operator2/2
  Logical Operator/1 -> Logical Operator2/1
  Compare To Constant/1 -> Logical Operator1/2
  Compare To Constant3/1 -> Logical Operator1/1
  Compare To Constant2/1 -> Logical Operator/2
  Compare To Constant1/1 -> Logical Operator/1
  LaneQlEC_stDvtThresActvFlg/1 -> Compare To Constant2/1, Compare To Constant3/1
  Data Type Conversion/1 -> LaneQlEC_stLaneQlECFlgLKA/1
  LaneQlEC_stFacmR0Ql/1 -> Compare To Constant1/1
  LaneQlEC_stFacmL0Ql/1 -> Compare To Constant/1

== system D53_LKAS/LL/LLOn/LL State Determination (LLStateDet)/LL State Machine Conditions (LLSMCon)/Deactivation Condition (DeactvC)/Deactivation Condition Synthesis (DeactvCSyn) ==
  DeactvCSyn_stDACMode : Inport
  DeactvCSyn_stDvtThresActvFlgLDW : Inport  Port=2
  DeactvCSyn_stDvtThresActvFlgLKA : Inport  Port=3
  DvrTkCon_stDvrTkConFlg : Inport  Port=4
  DeactvCSyn_stEPSCFlg : Inport  Port=5
  DeactvCSyn_stExitFlg : Inport  Port=6
  Cast To Single : DataTypeConversion  OutDataTypeStr=uint8
  Cast To Single1 : DataTypeConversion  OutDataTypeStr=uint8
  Default Flag (DflFlg) : Subsystem  TreatAsAtomicUnit=on
  Default Flag (DflFlg)1 : Subsystem  TreatAsAtomicUnit=on
  If : If  NumInputs=2  IfExpression=(u1 ==1|u1==2)& u2 == 0
  If1 : If  NumInputs=4  IfExpression=u1 == 2 & (u3 == 1 | u4 == 1)
  LDW Deactivation Flag (LDWDeactvFlg) : Subsystem  TreatAsAtomicUnit=on
  LKA Deactivation Flag (LKADeactvFlg) : Subsystem  TreatAsAtomicUnit=on
  Logical Operator : Logic  Operator=OR  AllPortsSameDT=off  OutDataTypeStr=boolean
  Merge : Merge
  Merge1 : Merge
  DeactvCSyn_stLDWDeactvCSyn : Outport
  DeactvCSyn_stLKADeactvCSyn : Outport  Port=2
  wires:
  DeactvCSyn_stDvtThresActvFlgLDW/1 -> If/2
  Logical Operator/1 -> Cast To Single/1
  DvrTkCon_stDvrTkConFlg/1 -> Logical Operator/1
  Cast To Single/1 -> If1/3
  If1/1 -> LKA Deactivation Flag (LKADeactvFlg)/Action
  Default Flag (DflFlg)1/1(Out) -> Merge1/2
  LKA Deactivation Flag (LKADeactvFlg)/1(Out) -> Merge1/1
  DeactvCSyn_stExitFlg/1 -> Cast To Single1/1
  DeactvCSyn_stEPSCFlg/1 -> Logical Operator/2
  Merge1/1 -> DeactvCSyn_stLKADeactvCSyn/1
  If1/2 -> Default Flag (DflFlg)1/Action
  Default Flag (DflFlg)/1(Out) -> Merge/2
  Merge/1 -> DeactvCSyn_stLDWDeactvCSyn/1
  DeactvCSyn_stDvtThresActvFlgLKA/1 -> If1/2
  DeactvCSyn_stDACMode/1 -> If/1, If1/1
  If/2 -> Default Flag (DflFlg)/Action
  If/1 -> LDW Deactivation Flag (LDWDeactvFlg)/Action
  LDW Deactivation Flag (LDWDeactvFlg)/1(Out) -> Merge/1
  Cast To Single1/1 -> If1/4

== system D53_LKAS/LL/LLOn/LL State Determination (LLStateDet)/LL State Machine Conditions (LLSMCon)/Deactivation Condition (DeactvC)/Deviation Threshold Condition (DvtThresCon) ==
  DvtThresCon_vVehSpd : Inport
  DvtThresCon_bsL0Info : Inport  Port=2
  DvtThresCon_bsR0Info : Inport  Port=3
  DvtThresCon_bsTTLCInfo : Inport  Port=4
  DvtThresCon_bsHdAgInfo : Inport  Port=5
  DvtThresCon_bsDvtThresClb : Inport  Port=6
  Active Lane Calculation (ActLanCalc) : Subsystem
  Bus Selector : BusSelector  OutputSignals=LftTTLC,RgtTTLC
  Bus Selector1 : BusSelector  OutputSignals=ActvCClb
  Bus Selector2 : BusSelector  OutputSignals=phiHdAgLft,phiHdAgRgt
  Deviation Calculation (DvtCalc) : Subsystem
  Deviation Speed Calculation (DvtSpdCalc) : Subsystem
  Deviation Threshold Judgement LDW (DvtThresJdg) : Subsystem
  Deviation Threshold Judgement LKA (DvtThresJdg) : Subsystem
  Saturation1 : Saturate  UpperLimit=1  LowerLimit=-1
  Saturation5 : Saturate  UpperLimit=1  LowerLimit=-1
  DvtThresCon_stDvtThresActvFlgLDW : Outport
  DvtThresCon_stDvtThresActvFlgLKA : Outport  Port=2
  wires:
  Saturation1/1 -> Deviation Threshold Judgement LDW (DvtThresJdg)/2(DvtThresJdg_lRgtDvt), Deviation Threshold Judgement LKA (DvtThresJdg)/2(DvtThresJdg_lRgtDvt)
  Bus Selector/1 -> Deviation Threshold Judgement LDW (DvtThresJdg)/5(DvtThresJdg_tiLftTTLC), Deviation Threshold Judgement LKA (DvtThresJdg)/5(DvtThresJdg_tiLftTTLC)  "<LftTTLC>"
  Saturation5/1 -> Deviation Threshold Judgement LDW (DvtThresJdg)/1(DvtThresJdg_lLftDvt), Deviation Threshold Judgement LKA (DvtThresJdg)/1(DvtThresJdg_lLftDvt)
  Deviation Speed Calculation (DvtSpdCalc)/2(DvtSpdCalc_vRgtDvtSpd) -> Deviation Threshold Judgement LDW (DvtThresJdg)/4(DvtThresJdg_vRgtDvtSpd), Deviation Threshold Judgement LKA (DvtThresJdg)/4(DvtThresJdg_vRgtDvtSpd)  "DvtSpdCalc_vRgtDvtSpd"
  Bus Selector/2 -> Deviation Threshold Judgement LDW (DvtThresJdg)/6(DvtThresJdg_tiRgtTTLC), Deviation Threshold Judgement LKA (DvtThresJdg)/6(DvtThresJdg_tiRgtTTLC)  "<RgtTTLC>"
  Deviation Speed Calculation (DvtSpdCalc)/1(DvtSpdCalc_vLftDvtSpd) -> Deviation Threshold Judgement LDW (DvtThresJdg)/3(DvtThresJdg_vLftDvtSpd), Deviation Threshold Judgement LKA (DvtThresJdg)/3(DvtThresJdg_vLftDvtSpd)  "DvtSpdCalc_vLftDvtSpd"
  Active Lane Calculation (ActLanCalc)/1(ActLanCalc_ActvCClbOut) -> Deviation Threshold Judgement LDW (DvtThresJdg)/7(DvtThresJdg_bsDvtThresClb), Deviation Threshold Judgement LKA (DvtThresJdg)/7(DvtThresJdg_bsDvtThresClb)
  Deviation Threshold Judgement LDW (DvtThresJdg)/1(DvtThresJdg_stDvtThresActvFlg) -> DvtThresCon_stDvtThresActvFlgLDW/1  "DvtThresActvFlg"
  Bus Selector2/2 -> Deviation Speed Calculation (DvtSpdCalc)/2(DvtSpdCalc_phiPrvwHdAgRgt)  "<phiHdAgRgt>"
  Bus Selector2/1 -> Deviation Speed Calculation (DvtSpdCalc)/1(DvtSpdCalc_phiPrvwHdAgLft)  "<phiHdAgLft>"
  DvtThresCon_bsHdAgInfo/1 -> Bus Selector2/1
  DvtThresCon_bsTTLCInfo/1 -> Bus Selector/1  "TTLCInfo"
  DvtThresCon_vVehSpd/1 -> Deviation Speed Calculation (DvtSpdCalc)/3(DvtSpdCalc_vVehSpd)
  DvtThresCon_bsDvtThresClb/1 -> Bus Selector1/1
  Deviation Threshold Judgement LKA (DvtThresJdg)/1(DvtThresJdg_stDvtThresActvFlg) -> DvtThresCon_stDvtThresActvFlgLKA/1  "DvtThresActvFlg"
  Deviation Calculation (DvtCalc)/2(DvtCalc_lRgtDvt) -> Saturation1/1  "DvtCalc_lRgtDvt"
  Deviation Calculation (DvtCalc)/1(DvtCalc_lLftDvt) -> Saturation5/1  "DvtCalc_lLftDvt"
  DvtThresCon_bsR0Info/1 -> Active Lane Calculation (ActLanCalc)/2(ActLanCalc_bsR0Info), Deviation Calculation (DvtCalc)/2(DvtCalc_bsR0Info)
  DvtThresCon_bsL0Info/1 -> Active Lane Calculation (ActLanCalc)/1(ActLanCalc_bsL0Info), Deviation Calculation (DvtCalc)/1(DvtCalc_bsL0Info)
  Bus Selector1/1 -> Active Lane Calculation (ActLanCalc)/3(ActLanCalc_ActvCClb)  "<ActvCClb>"
